simulink model "OCDC_model"  (R2021a)
settings: Solver=ode23t  StartTime=0.0  StopTime=25  FixedStep=0.0001  MaxStep=0.01  RelTol=1e-3
values from neighbouring files (symbols this model uses):
  boom_cylinder_A_area = pi * (boom_cylinder_cyl_diam / 2) ^2    (= 15393.8040026)    [condition_parameters.m]
  boom_cylinder_B_area = boom_cylinder_A_area - (boom_cylinder_rod_diam / 2) ^2    (= -24979606.446)    [condition_parameters.m]
  oomega_max = 4000    [OCDC_parameters.m]
  oomega_min = 750    [OCDC_parameters.m]
  spool_x_max = 10    [M1_32.m]
  U_max = 10    [OCDC_parameters.m]
  U_modeshift = 6    [OCDC_parameters.m]
undefined symbols (not defined in the file or in its folder): main_pump_disp, sigbuilder_block
libraries: SimscapeFluids_lib x13, nesl_utility x9, fl_lib x8, pid_lib x3, sh_lib x2
(part 2 of 2)

== matlab function OCDC_model/Motor controller (EHA) and mode selector/MATLAB Function2 ==
  data: U_1 input; U_2 input; oomega output; oomega_max input; oomega_min input; U_max input; U_modeshift input; EHA_mode output
%function [oomega_U, EHA_mode]= fcn(U_1, oomega_max, oomega_min, U_max, U_modeshift)
%
%k = (oomega_max - oomega_min)/(U_max-U_modeshift);
%
%
%if U_1<=-U_modeshift                                                    
%    oomega_U = -k*(U_1+U_max)+oomega_max;
%    EHA_mode = 1;
%elseif U_1>=U_modeshift
%    oomega_U = k*(U_1-U_max)+oomega_max;
%    EHA_mode = 1;
%else   
%    oomega_U = oomega_min;
%    EHA_mode = 0;
%end
%

function [oomega, EHA_mode]= fcn(U_1,U_2, oomega_max, oomega_min, U_max, U_modeshift)

k = (oomega_max - oomega_min*(1+abs(U_1*U_2)/U_modeshift))/(U_max-U_modeshift);
oomega_unlim = 500;

if U_1<=-U_modeshift                                  %1. sylinteri sisään DDH                             
    oomega_unlim = -k*(U_1+U_max)+oomega_max;
    EHA_mode = 1;
elseif U_1>=U_modeshift                               %1. sylinteri ulos DDH
    oomega_unlim = k*(U_1-U_max)+oomega_max;
    EHA_mode = 1;
else
    if U_2<=-U_modeshift                              %2. sylinteri sisään DDH
        oomega_unlim = -k*(U_2+U_max)+oomega_max;
        EHA_mode = 0;
    elseif U_2>=U_modeshift;                          %2. sylinteri ulos DDH
        oomega_unlim = k*(U_2-U_max)+oomega_max;
        EHA_mode = 0;
    else
        EHA_mode = 0;
        oomega_unlim = oomega_min*(1+abs(U_1*U_2)/U_modeshift);
    end
end

oomega = min(oomega_max, oomega_unlim);

end
